simulink model "BLAC_MotorCtrl_Math"  (R2023b)
settings: Solver=FixedStepDiscrete  StartTime=0.0  StopTime=0.1  FixedStep=MC_Sim_BaseStep  RelTol=1e-3  EnableMultiTasking=on
values from neighbouring files (symbols this model uses):
  MC_Hardware_Chip_ADCResultBit = 0.0    [MotorControlDataDictionary_Math.sldd]
  MC_Hardware_Chip_ADCVoltageMax = 1.0    [MotorControlDataDictionary_Math.sldd]
  MC_Hardware_Chip_ADCVoltageRefence = 0.0    [MotorControlDataDictionary_Math.sldd]
  MC_Hardware_Chip_CSAGain = 1.0    [MotorControlDataDictionary_Math.sldd]
  MC_Hardware_Sample_Resistor = 0.001    [MotorControlDataDictionary_Math.sldd]
  MC_MotorModel_Machine_Damp = 0.0    [MotorControlDataDictionary_Math.sldd]
  MC_MotorModel_Machine_Ineria = 0.0    [MotorControlDataDictionary_Math.sldd]
  MC_MotorModel_Machine_Tfric = 0.0    [MotorControlDataDictionary_Math.sldd]
  MC_MotorModel_Rotor_Pn = 4.0    [MotorControlDataDictionary_Math.sldd]
  MC_MotorModel_Stator_Ld = 0.0    [MotorControlDataDictionary_Math.sldd]
  MC_MotorModel_Stator_Lq = 0.0    [MotorControlDataDictionary_Math.sldd]
  MC_MotorModel_Stator_Rs = 1.0    [MotorControlDataDictionary_Math.sldd]
  MC_Sim_BaseStep = 2.5E-8    [MotorControlDataDictionary_Math.sldd]
  MC_Sim_HFTStep = 6.6675E-5    [MotorControlDataDictionary_Math.sldd]
undefined symbols (not defined in the file or in its folder): MC_MOS_DeadTime, MC_Motor_Phi, MC_Motor_Rotor_Pn, MC_Motor_Stator_Ld, MC_Motor_Stator_Lq, MC_Motor_Stator_Rs, MC_Param_CurrentPI_Ki, MC_Param_CurrentPI_Kp, MC_Param_CurrentPI_UdInteMax, MC_Param_CurrentPI_UdInteMin, MC_Param_CurrentPI_UdMax, MC_Param_CurrentPI_UdMin, MC_Param_CurrentPI_UqInteMax, MC_Param_CurrentPI_UqInteMin, MC_Param_CurrentPI_UqMax, MC_Param_CurrentPI_UqMin, MC_Param_Flux_Gamma, MC_Param_Flux_Lalpha, MC_Param_Flux_Lbeta, MC_Param_Flux_Ralpha, MC_Param_Flux_Rbeta, MC_Param_Luen_BEMFalpha, MC_Param_Luen_BEMFbeta, MC_Param_Luen_BEMFErr, MC_Param_Luen_Currentalpha, MC_Param_Luen_Currentbeta, MC_Param_Luen_CurrentErr, MC_Param_Luen_PLL_Ki, MC_Param_Luen_PLL_Kp, MC_Param_Luen_Voltagealpha, MC_Param_Luen_Voltagebeta, MC_Param_PhasetoReal, MC_Param_SMO_CoffA, MC_Param_SMO_CoffB, MC_Param_SpeedtoTheta, MC_Param_SVPWM_DutyMax, MC_Param_SVPWM_DutyMin, MC_Param_SVPWM_SampleOffset1, MC_Param_SVPWM_SampleOffset2, MC_Param_SVPWM_SampleValid
libraries: simulink x29, spsSeriesRLCBranchLib x6, spsVoltageMeasurementLib x6, spsIGBTLib x6, spsDiodeLib x4, spsACVoltageSourceLib x1, spsGroundLib x1, spsPermanentMagnetSynchronousMachineLib x1, spsThreePhaseVIMeasurementLib x1, spspowerguiLib x1
(part 1 of 3)
settings Model: DataDictionary=MotorControlDataDictionary_Math.sldd  SimulationMode=accelerator  Creator=YXuan  LastModifiedBy=YXuan
settings SolverCC: PositivePriorityOrder=on
settings OptimizationCC: DefaultParameterBehavior=Inlined  EnhancedBackFolding=on  PassReuseOutputArgsAs=Individual arguments  ZeroExternalMemoryAtStartup=off  ZeroInternalMemoryAtStartup=off  OptimizeBlockOrder=speed  DifferentSizesBufferReuse=on  OptimizationCustomize=off  EfficientTunableParamExpr=on
settings DebuggingCC: ParameterTunabilityLossMsg=error
settings SFSimCC: MATLABDynamicMemAlloc=off
settings RTWCC: Description=Embedded Coder  SystemTargetFile=ert.tlc  TemplateMakefile=ert_default_tmf
settings CodeAppCC: ForceParamTrailComments=on  IgnoreCustomStorageClasses=off  OperatorAnnotations=on  SimulinkDataObjDesc=on  SFDataObjDesc=on  InsertBlockDesc=on
settings ERTTargetCC: TargetLangStandard=C99 (ISO)  GenerateSampleERTMain=on  InlinedParameterPlacement=NonHierarchical  ERTCustomFileTemplate=example_file_process.tlc

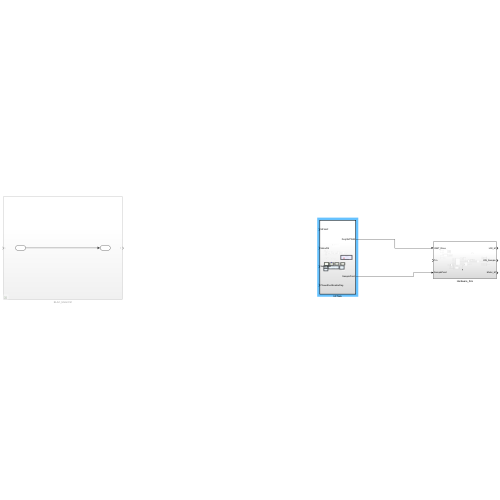
[thumbnail: Simulink's stored preview of the top-level diagram]
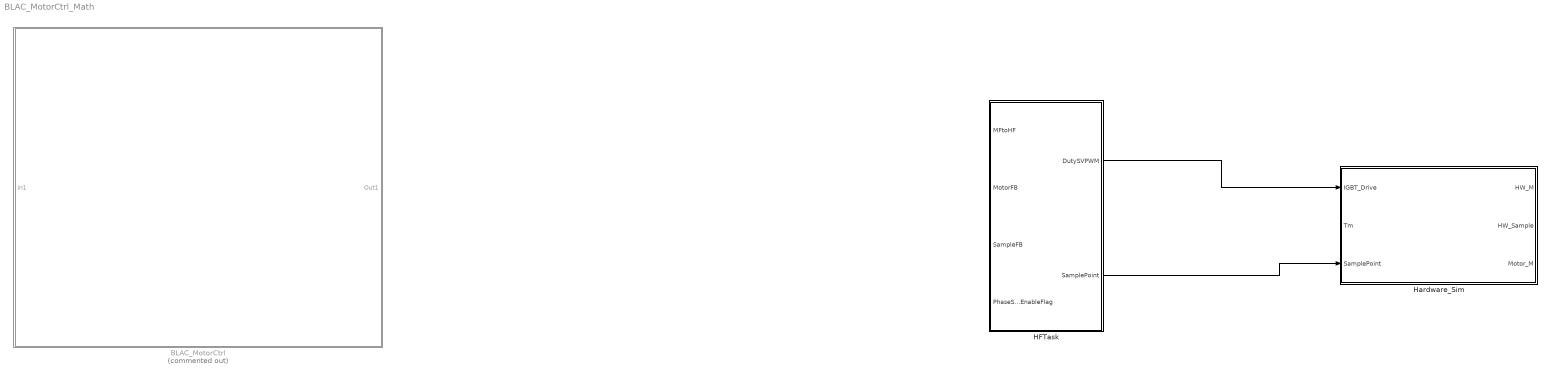
== system BLAC_MotorCtrl_Math ==
  BLAC_MotorCtrl : Subsystem  Commented=on
  HFTask : Subsystem  TreatAsAtomicUnit=on  SystemSampleTime=MC_Sim_HFTStep
  Hardware_Sim : Subsystem
  wires:
  HFTask/1(DutySVPWM) -> Hardware_Sim/1(IGBT_Drive)
  HFTask/2(SamplePoint) -> Hardware_Sim/3(SamplePoint)

== system BLAC_MotorCtrl_Math/BLAC_MotorCtrl ==
  In1 : Inport
  Out1 : Outport
  wires:
  In1/1 -> Out1/1

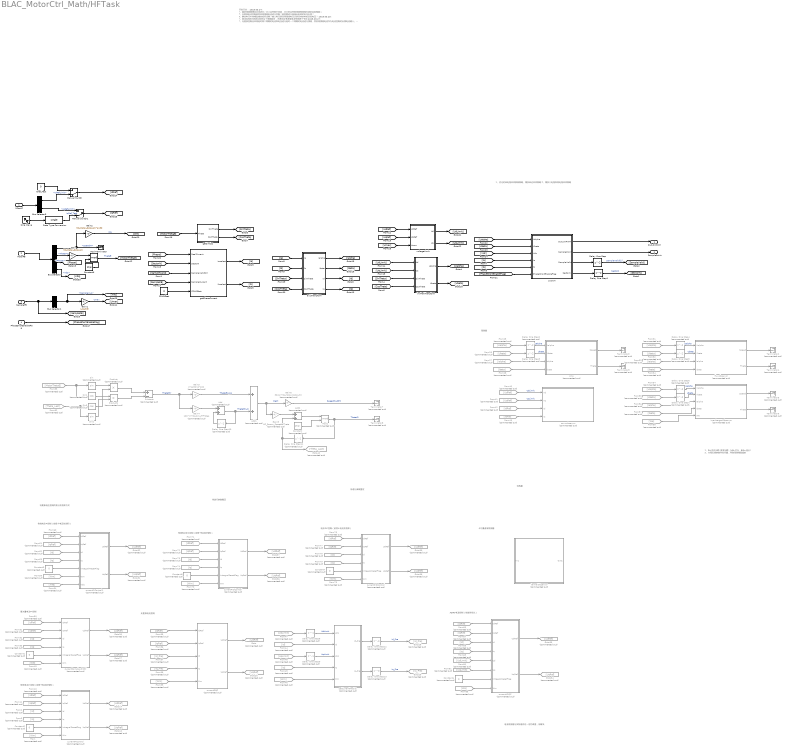
== system BLAC_MotorCtrl_Math/HFTask ==
  note: 待更新电压控制的积分抗饱和方式
  note: 传统电流PI控制（前馈+电流抗饱和）
  note: 1、PLL存在问题(带宽问题，10hz可以，50hz溢出)
      | 2、方程反馈参数存在问题，导致观测角度超前
  note: 观测器
  note: 无差拍电流控制
  note: 开发日志：
      | 2025.03.24:
      | 1、磁链观测器增益应该适中（过小会导致不收敛，过大则会导致观测角度相位超前实际角度）
      | 2、无差拍电流控制是否采用预测电流进行控制？是否要进行旋转反电势的电压补偿？
      | 3、静态电压补偿模型增益如何设置？输入电压是采用理想电压还是采样的电机实际电压？
      | 2025.03.25:
      | 1、测试发现电压和电流呈现2个周期延时，无差拍应考虑做电流预测两个节拍
      | 2025.03.27：
      | 1、无差拍控制应采用延时两个周期的电流和电压进行延时一个周期的电流进行预测，然后用预测电流作为电流控制的反馈电流输入。
      | 2025.12.13:
      | 1、增加真实相电压计算（待添加）
      | 2、考虑MPTA、弱磁、以及MPTV模块的防止位置
      | 2026.01.01：
      | 1、增加卡尔曼滤波模块（未构建）
      | 2、增加PIR控制器（未整定参数）
      | 2026.01.28：
      | 1、发现ADRC的电流观测值初期收敛速度较慢，并且存在稳定的误差。
  note: 复矢量电流PI控制
  note: 传统电流PI控制（前馈+电压抗饱和）
  note: ADRC电流控制（性能待优化）
  note: 传统电流PID控制（前馈+电流抗饱和）
  note: 待进行参数整定
  note: 电流PIR控制（前馈+电流抗饱和）
  note: 待进行参数整定
  note: 卡尔曼滤波观测器
  note: 待构建
  note: 1、优化的单电阻采样移相策略、增加单边采样策略
      | 2、增加三电阻和两电阻采样策略
  note: 电流观测值与实际值存在一定的误差，待解决
  MFtoHF : Inport
  MotorFB : Inport  Port=2
  SampleFB : Inport  Port=3
  PhaseShortEnableFlag : Inport  Port=4
  Add : Sum  Commented=on
  Add1 : Sum  Commented=on
  Add2 : Sum  Commented=on
  Bus Selector : BusSelector  OutputSignals=SpeedM,ThetaM,PhaseI,Vdq
  Bus Selector1 : BusSelector  OutputSignals=SampleVus
  Bus Selector3 : BusSelector  OutputSignals=IdRefLimit,IqRefLimit
  CSAOffset : Constant  Value=0  OutDataTypeStr=single
  Constant : Constant  Commented=on  Value=2*pi  OutDataTypeStr=single
  Constant{1..5,7} (6 alike) : Constant  Commented=on  Value=0  OutDataTypeStr=boolean
  Constant6 : Constant  Value=2*pi  OutDataTypeStr=single
  Data Type Conversion : DataTypeConversion  OutDataTypeStr=single  RndMeth=Simplest  SaturateOnIntegerOverflow=off
  Delay One Step : Delay
  Delay One Step1 : Delay
  Delay One Step{8..11} (4 alike) : Delay  Commented=on  DelayLength=1
  Delay One Step12 : Delay  Commented=on  DelayLength=0
  Delay One Step13 : Delay  Commented=on  DelayLength=0
  Delay One Step{2..7} (6 alike) : Delay  Commented=on
  From{,39,46,59,70,75} (6 alike) : From  Commented=on  GotoTag=Wm
  From{10,35,42,50,60,66,71,76} (8 alike) : From  Commented=on  GotoTag=IdRef
  From{11,36,43,51,61,67,72,77} (8 alike) : From  Commented=on  GotoTag=IqRef
  From{2,44,52,62,68,73,78} (7 alike) : From  Commented=on  GotoTag=Id
  From25 : From  Commented=on  GotoTag=Ualpha
  From26 : From  Commented=on  GotoTag=Ubeta
  From27 : From  Commented=on  GotoTag=Ialpha
  From28 : From  Commented=on  GotoTag=Ibeta
  From{3,45,53,63,69,74,79} (7 alike) : From  Commented=on  GotoTag=Iq
  From31 : From  Commented=on  GotoTag=Ualpha
  From32 : From  Commented=on  GotoTag=Ubeta
  From33 : From  Commented=on  GotoTag=Ialpha
  From34 : From  Commented=on  GotoTag=Ibeta
  From37 : From  Commented=on  GotoTag=Id_Pre
  From38 : From  Commented=on  GotoTag=Iq_Pre
  From40 : From  Commented=on  GotoTag=UdRef
  From41 : From  Commented=on  GotoTag=UqRef
  From47 : From  Commented=on  GotoTag=UdLimit
  From48 : From  Commented=on  GotoTag=UqLimit
  From49 : From  Commented=on  GotoTag=We
  From54 : From  Commented=on  GotoTag=Ualpha
  From55 : From  Commented=on  GotoTag=Ubeta
  From56 : From  Commented=on  GotoTag=Ialpha
  From57 : From  Commented=on  GotoTag=Ibeta
  From58 : From  Commented=on  GotoTag=We
  From64 : From  Commented=on  GotoTag=Vdq
  From65 : From  Commented=on  GotoTag=We
  From80 : From  Commented=on  GotoTag=UdLimit
  From81 : From  Commented=on  GotoTag=UqLimit
  From82 : From  Commented=on  GotoTag=Theta_Last
  From83 : From  Commented=on  GotoTag=MotorThetaE
  Gain : Gain  Gain=MC_Motor_Rotor_Pn  OutDataTypeStr=single
  Gain1 : Gain  Gain=1/sqrt(3)  OutDataTypeStr=single
  Gain2 : Gain  Gain=MC_Motor_Rotor_Pn*pi/30
  Gain3 : Gain  Commented=on  Gain=2*sqrt(2)/2*100
  Gain4 : Gain  Commented=on  Gain=100^2*MC_Sim_HFTStep
  Gain5 : Gain  Commented=on  Gain=MC_Param_SpeedtoTheta  OutDataTypeStr=single  RndMeth=Simplest
  Gain6 : Gain  Commented=on  Gain=30/(pi*MC_Motor_Rotor_Pn)  OutDataTypeStr=single  RndMeth=Simplest
  Goto{,14,30,32,35,37,39} (7 alike) : Goto  Commented=on  GotoTag=UdRef
  Goto{10,26..27,31,34,36,38} (7 alike) : Goto  Commented=on  GotoTag=UqRef
  Goto28 : Goto  Commented=on  GotoTag=Id_Pre
  Goto29 : Goto  Commented=on  GotoTag=Iq_Pre
  Goto40 : Goto  Commented=on  GotoTag=Theta_Last
  Idref_Test : Constant  Value=0  OutDataTypeStr=single
  LuenbergerObservor : Subsystem  Commented=on
  Manual Switch : ManualSwitch  CurrentSetting=0
  Manual Switch1 : ManualSwitch  CurrentSetting=0
  Mod : Math  Operator=mod
  Mod1 : Math  Commented=on  Operator=mod
  Product : Product  Commented=on
  Product1 : Product  Commented=on
  Sin : Trigonometry  Commented=on  OutputSignalType=real
  Sin1 : Trigonometry  Commented=on  Operator=cos  OutputSignalType=real
  Sin2 : Trigonometry  Commented=on  OutputSignalType=real
  Sin3 : Trigonometry  Commented=on  Operator=cos  OutputSignalType=real
  Sine Wave : Sin  Amplitude=20  Frequency=2*pi*1  SampleTime=MC_Sim_HFTStep
  Subtract : Sum  Commented=on  Inputs=+-
  Terminator : Terminator
  Terminator{1..8} (8 alike) : Terminator  Commented=on
  axisTransform : Subsystem
  currentADRC : Subsystem  Commented=on
  currentComplexPICtrl : Subsystem  Commented=on
  currentDBC : Subsystem  Commented=on
  currentPIControl : Subsystem  Commented=on
  currentPIControl1 : Subsystem  Commented=on
  currentPIDControl : Subsystem  Commented=on
  currentPIRControl : Subsystem  Commented=on
  fluxobservor : Subsystem  Commented=on
  getCurrentPredict : Subsystem  Commented=on
  getPhaseCurrent : Subsystem
  getSinCos : Subsystem
  invParkTransform : Subsystem
  karmalObservor : Subsystem  Commented=on
  scvmobservor : Subsystem  Commented=on
  smo : Subsystem  Commented=on
  svpwm : Subsystem  TreatAsAtomicUnit=on
  voltageLimit : Subsystem
  DutySVPWM : Outport
  SamplePoint : Outport  Port=2
  wires:
  MFtoHF/1 -> Bus Selector3/1
  Delay One Step2/1 -> smo/1(Valpha)  "Ualpha"
  From25/1 -> Delay One Step2/1
  Delay One Step3/1 -> smo/2(Vbeta)  "Ubeta"
  From26/1 -> Delay One Step3/1
  From27/1 -> smo/3(Ialpha)
  From28/1 -> smo/4(Ibeta)
  smo/1(Speed) -> Terminator2/1
  smo/2(Theta) -> Terminator3/1
  [PhaseShortEnableFlag] -> svpwm/6(PhaseShortEnableFlag)
  [Umax] -> voltageLimit/3(Umax)
  svpwm/4(SectorN) -> Delay One Step1/1
  axisTransform/2(Ibeta) -> [Ibeta]
  svpwm/3(SampleValid) -> Delay One Step/1
  svpwm/1(DutySVPWM) -> DutySVPWM/1
  [SampleFB] -> getPhaseCurrent/4(SampleCurrent)
  [SectorN] -> getPhaseCurrent/2(SectorN)
  [UdRef] -> voltageLimit/1(UdRef)
  [UdLimit] -> invParkTransform/1(Ud)
  currentPIControl/1(UdRef) -> Goto14/1
  [Ubeta] -> svpwm/2(Vbeta)
  axisTransform/1(Ialpha) -> [Ialpha]
  [UqRef] -> voltageLimit/2(UqRef)
  [Ualpha] -> svpwm/1(Valpha)
  [Ia] -> axisTransform/1(Ia)
  svpwm/2(SamplePoint) -> SamplePoint/1
  currentPIControl/2(UqRef) -> Goto10/1
  [Vdc] -> svpwm/3(Vdc)
  voltageLimit/1(Ud) -> [UdLimit]
  [MotorThetaE] -> getSinCos/1(Theta)
  From2/1 -> currentPIControl/3(Id)
  getSinCos/1(SinTheta) -> [SinTheta]
  [SampleValid] -> getPhaseCurrent/3(SampleValid[2])
  axisTransform/3(Id) -> [Id]
  getPhaseCurrent/2(Ibselect) -> [Ib]
  From/1 -> currentPIControl/6(Wm)
  axisTransform/4(Iq) -> [Iq]
  From3/1 -> currentPIControl/4(Iq)
  Constant2/1 -> currentPIControl/5(IntregralResetFlag)
  [Ib] -> axisTransform/2(Ib)
  [UqLimit] -> invParkTransform/2(Uq)
  [SinTheta] -> invParkTransform/3(SinTheta)
  Delay One Step1/1 -> [SectorN]  "SectorN"
  [CosTheta] -> invParkTransform/4(CosTheta)
  [PhaseI] -> getPhaseCurrent/1(RealCurrent)
  invParkTransform/1(Ualpha) -> [Ualpha]
  Delay One Step/1 -> [SampleValid]  "SampleValid[2]"
  getSinCos/2(CosTheta) -> [CosTheta]
  voltageLimit/2(Uq) -> [UqLimit]
  [SinTheta] -> axisTransform/3(SinTheta)
  getPhaseCurrent/1(Iaselect) -> [Ia]
  CSAOffset/1 -> getPhaseCurrent/5(CSAOffset)
  [CosTheta] -> axisTransform/4(CosTheta)
  invParkTransform/2(Ubeta) -> [Ubeta]
  [Ib] -> svpwm/5(Ib)
  [Ia] -> svpwm/4(Ia)
  Bus Selector/2 -> Gain/1  "<ThetaM>"
  PhaseShortEnableFlag/1 -> [PhaseShortEnableFlag]
  Bus Selector/1 -> Terminator/1, Gain2/1  "<SpeedM>"
  Mod/1 -> [MotorThetaE]  "ThetaE"
  Bus Selector/3 -> [PhaseI]  "<PhaseI>"
  Gain/1 -> Mod/1
  Bus Selector1/1 -> [Vdc], Gain1/1  "<SampleVus>"
  SampleFB/1 -> [SampleFB], Bus Selector1/1
  Gain1/1 -> [Umax]  "Umax"
  Constant6/1 -> Mod/2
  MotorFB/1 -> Bus Selector/1
  From10/1 -> currentPIControl/1(IdRef)
  From11/1 -> currentPIControl/2(IqRef)
  From34/1 -> fluxobservor/4(Ibeta)
  From33/1 -> fluxobservor/3(Ialpha)
  From32/1 -> Delay One Step5/1
  From31/1 -> Delay One Step4/1
  Delay One Step4/1 -> fluxobservor/1(Valpha)  "Ualpha"
  Delay One Step5/1 -> fluxobservor/2(Vbeta)  "Ubeta"
  fluxobservor/1(Speed) -> Terminator1/1
  fluxobservor/2(Theta) -> Terminator4/1
  currentDBC/2(UqRef) -> Goto26/1
  From36/1 -> currentDBC/2(IqRef)
  From35/1 -> currentDBC/1(IdRef)
  From37/1 -> currentDBC/3(Id)
  From38/1 -> currentDBC/4(Iq)
  From39/1 -> currentDBC/5(Wm)
  From41/1 -> scvmobservor/2(Vq)  "UqLimit"
  From40/1 -> scvmobservor/1(Vd)  "UdLimit"
  From42/1 -> scvmobservor/3(Id)
  From43/1 -> scvmobservor/4(Iq)
  Gain2/1 -> [We]  "We"
  From44/1 -> getCurrentPredict/2(Id)
  From45/1 -> getCurrentPredict/4(Iq)
  From46/1 -> getCurrentPredict/5(Wm)
  From47/1 -> Delay One Step8/1
  From48/1 -> Delay One Step9/1
  getCurrentPredict/1(Id_Pre) -> Delay One Step12/1
  getCurrentPredict/2(Iq_Pre) -> Delay One Step13/1
  currentDBC/1(UdRef) -> Goto/1
  Delay One Step8/1 -> getCurrentPredict/1(Ud1)  "UdLimit"
  Delay One Step9/1 -> getCurrentPredict/3(Uq1)  "UqLimit"
  Delay One Step12/1 -> Goto28/1  "Id_Pre"
  Delay One Step13/1 -> Goto29/1  "Iq_Pre"
  From51/1 -> currentComplexPICtrl/2(IqRef)
  From50/1 -> currentComplexPICtrl/1(IdRef)
  Constant1/1 -> currentComplexPICtrl/5(IntregralResetFlag)
  From53/1 -> currentComplexPICtrl/4(Iq)
  From49/1 -> currentComplexPICtrl/6(Wm)
  From52/1 -> currentComplexPICtrl/3(Id)
  currentComplexPICtrl/2(UqRef) -> Goto27/1
  currentComplexPICtrl/1(UdRef) -> Goto30/1
  LuenbergerObservor/1(Speed) -> Terminator5/1
  LuenbergerObservor/2(Theta) -> Terminator6/1
  From57/1 -> LuenbergerObservor/4(Ibeta)
  From56/1 -> LuenbergerObservor/3(Ialpha)
  From55/1 -> Delay One Step7/1
  From54/1 -> Delay One Step6/1
  Delay One Step7/1 -> LuenbergerObservor/2(Vbeta)  "Ubeta"
  Delay One Step6/1 -> LuenbergerObservor/1(Valpha)  "Ualpha"
  From58/1 -> LuenbergerObservor/5(We)
  From61/1 -> currentPIControl1/2(IqRef)
  From60/1 -> currentPIControl1/1(IdRef)
  Constant3/1 -> currentPIControl1/5(IntregralResetFlag)
  From63/1 -> currentPIControl1/4(Iq)
  From59/1 -> currentPIControl1/6(Wm)
  From62/1 -> currentPIControl1/3(Id)
  currentPIControl1/2(UqRef) -> Goto31/1
  currentPIControl1/1(UdRef) -> Goto32/1
  Bus Selector/4 -> [Vdq]  "<Vdq>"
  From64/1 -> currentPIControl1/7(Vdq)
  currentADRC/1(UdRef) -> Goto35/1
  currentADRC/2(UqRef) -> Goto34/1
  From68/1 -> currentADRC/3(Id)
  From65/1 -> currentADRC/8(Wm)
  From69/1 -> currentADRC/4(Iq)
  Constant4/1 -> currentADRC/7(IntregralResetFlag)
  From66/1 -> currentADRC/1(IdRef)
  From67/1 -> currentADRC/2(IqRef)
  Constant5/1 -> currentPIDControl/5(IntregralResetFlag)
  From71/1 -> currentPIDControl/1(IdRef)
  currentPIDControl/1(UdRef) -> Goto37/1
  From73/1 -> currentPIDControl/3(Id)
  From72/1 -> currentPIDControl/2(IqRef)
  currentPIDControl/2(UqRef) -> Goto36/1
  From70/1 -> currentPIDControl/6(Wm)
  From74/1 -> currentPIDControl/4(Iq)
  Bus Selector3/1 -> Manual Switch/2  "<IdRefLimit>"
  Bus Selector3/2 -> Manual Switch1/1  "<IqRefLimit>"
  Sine Wave/1 -> Data Type Conversion/1
  Manual Switch/1 -> [IdRef]
  Idref_Test/1 -> Manual Switch/1
  Manual Switch1/1 -> [IqRef]
  Data Type Conversion/1 -> Manual Switch1/2  "IqRef_Test"
  From79/1 -> currentPIRControl/4(Iq)
  From75/1 -> currentPIRControl/6(Wm)
  currentPIRControl/2(UqRef) -> Goto38/1
  From77/1 -> currentPIRControl/2(IqRef)
  From78/1 -> currentPIRControl/3(Id)
  currentPIRControl/1(UdRef) -> Goto39/1
  From76/1 -> currentPIRControl/1(IdRef)
  Constant7/1 -> currentPIRControl/5(IntregralResetFlag)
  From80/1 -> currentADRC/5(Ud)
  From81/1 -> currentADRC/6(Uq)
  Gain5/1 -> Add2/1
  Delay One Step10/1 -> Add/2
  Constant/1 -> Mod1/2
  Mod1/1 -> Terminator8/1, Delay One Step11/1  "ThetaPI"
  Delay One Step11/1 -> Goto40/1, Add2/2
  Gain3/1 -> Add1/1  "ThetaErr_Kp"
  Add1/1 -> Gain6/1, Gain5/1  "WePI"
  Add2/1 -> Mod1/1
  Gain6/1 -> Terminator7/1  "SpeedPI_RPM"
  Subtract/1 -> Gain3/1, Gain4/1  "ThetaErr"
  Add/1 -> Add1/2, Delay One Step10/1  "ThetaErr_Ki"
  Gain4/1 -> Add/1
  From83/1 -> Sin1/1, Sin/1
  From82/1 -> Sin2/1, Sin3/1
  Sin/1 -> Product/1
  Sin3/1 -> Product/2
  Product/1 -> Subtract/1
  Sin1/1 -> Product1/1
  Sin2/1 -> Product1/2
  Product1/1 -> Subtract/2

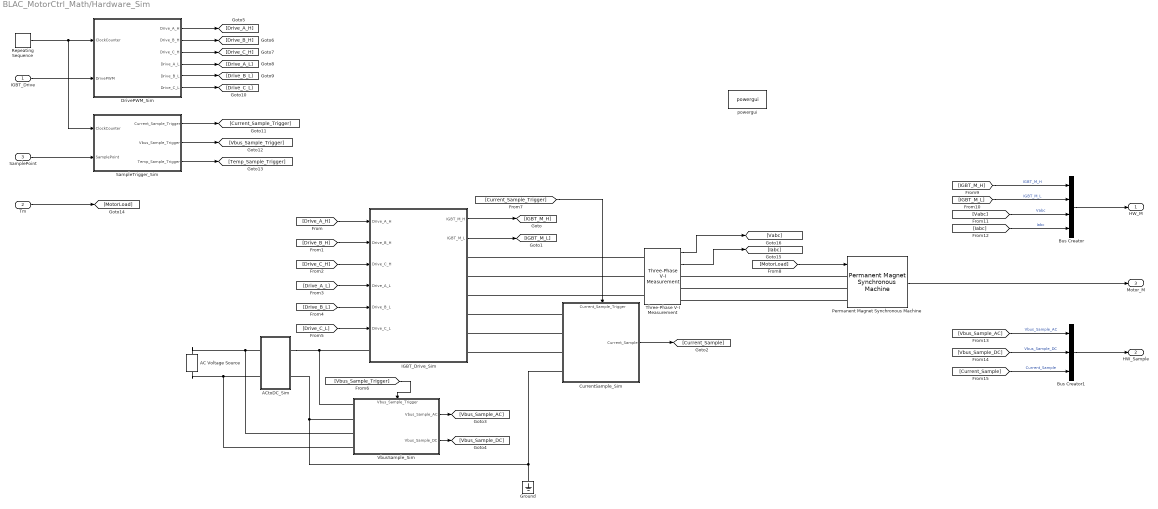
== system BLAC_MotorCtrl_Math/Hardware_Sim ==
  IGBT_Drive : Inport
  Tm : Inport  Port=2
  SamplePoint : Inport  Port=3
  AC Voltage Source : spsACVoltageSourceLib/AC Voltage Source  Amplitude=220*sqrt(2)  Phase=0  Frequency=50  SampleTime=-1  Measurements=None  BusType=swing  Pref=10e3  Qref=0  Qmin=-inf  Qmax=+inf
  ACtoDC_Sim : Subsystem
  Bus Creator : BusCreator  Inputs=4
  Bus Creator1 : BusCreator  Inputs=3
  CurrentSample_Sim : Subsystem
      settings: PortSchema="{\"entries\":[{\"content\":{\"sides\":[{\"content\":{\"connectorIds\":[\"LConn1\",\"LConn2\",\"LConn3\",\"LConn4\"]},\"type\":\"ConnectorPlacement.EquallySpacedRectSide\",\"uuid\":\"6ff7a8d3-c405-46c2-bb14-4046cb7aeae7\"},{\"content\":{\"connectorIds\":[\"Out1\"],\"side\":\"RIGHT\"},\"type\":\"ConnectorPlacement.EquallySpacedRectSide\",\"uuid\":\"30142a9b-9a7e-41fc-b1d2-e3039139c6ca\"},{\"content\":{\"connectorIds\":[\"In1\"],\"side\":\"TOP\"},\"type\":\"ConnectorPlacement.EquallySpacedRectSide\",\"uuid\":\"3160108e-a18c-4d1a-9078-164fb8c05fb9\"}]},\"type\":\"ConnectorPlacement.EquallySpacedConnector\",\"uuid\":\"b4e632a6-7f3d-4ba3-a4f0-ad8004e8ab56\"}],\"packageUris\":[\"http://schema.mathworks.com/mf0/Connector/R2020b\"],\"version\":\"1.0\"}"
  DrivePWM_Sim : Subsystem
  Ground : spsGroundLib/Ground  LConnTagsString=a
  IGBT_Drive_Sim : Subsystem
  Permanent Magnet Synchronous Machine : spsPermanentMagnetSynchronousMachineLib/Permanent Magnet Synchronous Machine  NbPhases=3  FluxDistribution=Sinusoidal  RotorType=Salient-pole  MechanicalLoad=Torque Tm  PresetModel=No  ShowDetailedParameters=on  MeasurementBus=on  Resistance=MC_MotorModel_Stator_Rs  Inductance=8.5e-3  dqInductances=[MC_MotorModel_Stator_Ld,MC_MotorModel_Stator_Lq]  La=0.000395  MachineConstant=Voltage Constant (V_peak L-L / krpm)  Flux=0  VoltageCst=MC_MotorModel_Magentic_Ke  TorqueCst=0  Flat=120  Mechanical=[MC_MotorModel_Machine_Ineria,MC_MotorModel_Machine_Damp,MC_MotorModel_Rotor_Pn,MC_MotorModel_Machine_Tfric]  PolePairs=4  InitialConditions=[0,0, 0,0]  InitialConditions5ph=[0 0 0 0 0 0]  RefAngle=Aligned with phase A axis (original Park)  IterativeDiscreteModel=Trapezoidal non iterative  TsBlock=-1  TsPowergui=0
  Repeating Sequence : simulink/Sources/Repeating Sequence  rep_seq_t=[0 MC_Sim_HFTStep/2 MC_Sim_HFTStep]  rep_seq_y=[0 1 0]
  SampleTrigger_Sim : Subsystem
  Three-Phase V-I Measurement : spsThreePhaseVIMeasurementLib/Three-Phase V-I Measurement  VoltageMeasurement=phase-to-ground  SetLabelV=off  LabelV=Vabc  Vpu=off  VpuLL=off  CurrentMeasurement=yes  SetLabelI=off  LabelI=Iabc  Ipu=off  Pbase=100e6  Vbase=500e3  OutputType=Complex  PhasorSimulation=off  PSBequivalent=0
  VbusSample_Sim : Subsystem
      settings: PortSchema="{\"entries\":[{\"content\":{\"sides\":[{\"content\":{\"connectorIds\":[\"LConn1\",\"LConn2\",\"LConn3\",\"LConn4\"]},\"type\":\"ConnectorPlacement.EquallySpacedRectSide\",\"uuid\":\"516f667a-d28d-4d7e-bf09-1844ec397ca8\"},{\"content\":{\"connectorIds\":[\"Out1\",\"Out2\"],\"side\":\"RIGHT\"},\"type\":\"ConnectorPlacement.EquallySpacedRectSide\",\"uuid\":\"8e4c85e3-3d11-4eb4-88a0-2693c28d829e\"},{\"content\":{\"connectorIds\":[\"In1\"],\"side\":\"TOP\"},\"type\":\"ConnectorPlacement.EquallySpacedRectSide\",\"uuid\":\"147b6efa-5ce1-4794-b48d-7dda172e67f0\"}]},\"type\":\"ConnectorPlacement.EquallySpacedConnector\",\"uuid\":\"ecacdeaf-2c45-44a5-a2ad-63e6b49d0bd0\"}],\"packageUris\":[\"http://schema.mathworks.com/mf0/Connector/R2020b\"],\"version\":\"1.0\"}"
  powergui : spspowerguiLib/powergui  Priority=1  SimulationMode=Discrete  SampleTime=MC_Sim_BaseStep  frequency=60  Iterations=50  frequencyindice=50  Pbase=100e6  ErrMax=1e-4  UnitsV=kV  UnitsW=MW  buscounter=0  FunctionMessages=off  echomessages=off  EnableUseOfTLC=off  CurrentSourceSwitches=off  DisableSnubberDevices=off  DisableRonSwitches=off  DisableVfSwitches=off  DisplayEquations=off  AutomaticDiscreteSolvers=off  SolverType=Tustin/Backward Euler (TBE)  Interpol=off  ExternalGateDelay=off  methode=off  Ts=100  x0status=blocks  SPID=on  SwTol=0  HookPort=off  NonlinearTolerance=1e-4  nMaxIteration=100  ContinueOnMaxIteration=off  RestoreLinks=warning  ResistiveCurrentMeasurement=off  Frange=[0:2:500]  Ylog=off  Xlog=on  ShowGrid=off  save=off  variable=ZData  structure=0  ZoomFFT=off  StartTime=0.0  cycles=1  DisplayStyle=1  fundamental=60  FreqAxis=off  MaxFrequency=1000  frequencyindicesteady=1  RmsSteady=1  display=off
  HW_M : Outport
  HW_Sample : Outport  Port=2
  Motor_M : Outport  Port=3
  wires:
  Permanent Magnet Synchronous Machine/1 -> Motor_M/1
  IGBT_Drive_Sim/1(IGBT_M_H) -> [IGBT_M_H]
  IGBT_Drive_Sim/2(IGBT_M_L) -> [IGBT_M_L]
  CurrentSample_Sim/1(Current_Sample) -> [Current_Sample]
  VbusSample_Sim/1(Vbus_Sample_AC) -> [Vbus_Sample_AC]
  VbusSample_Sim/2(Vbus_Sample_DC) -> [Vbus_Sample_DC]
  SamplePoint/1 -> SampleTrigger_Sim/2(SamplePoint)
  Repeating Sequence/1 -> SampleTrigger_Sim/1(ClockCounter), DrivePWM_Sim/1(ClockCounter)
  IGBT_Drive/1 -> DrivePWM_Sim/2(DrivePWM)
  DrivePWM_Sim/1(Drive_A_H) -> [Drive_A_H]
  DrivePWM_Sim/2(Drive_B_H) -> [Drive_B_H]
  DrivePWM_Sim/6(Drive_C_L) -> [Drive_C_L]
  DrivePWM_Sim/5(Drive_B_L) -> [Drive_B_L]
  DrivePWM_Sim/4(Drive_A_L) -> [Drive_A_L]
  DrivePWM_Sim/3(Drive_C_H) -> [Drive_C_H]
  SampleTrigger_Sim/1(Current_Sample_Trigger) -> [Current_Sample_Trigger]
  SampleTrigger_Sim/2(Vbus_Sample_Trigger) -> [Vbus_Sample_Trigger]
  SampleTrigger_Sim/3(Temp_Sample_Trigger) -> [Temp_Sample_Trigger]
  [Drive_A_H] -> IGBT_Drive_Sim/1(Drive_A_H)
  [Drive_B_H] -> IGBT_Drive_Sim/2(Drive_B_H)
  [Drive_C_H] -> IGBT_Drive_Sim/3(Drive_C_H)
  [Drive_A_L] -> IGBT_Drive_Sim/4(Drive_A_L)
  [Drive_B_L] -> IGBT_Drive_Sim/5(Drive_B_L)
  [Drive_C_L] -> IGBT_Drive_Sim/6(Drive_C_L)
  [Vbus_Sample_Trigger] -> VbusSample_Sim/1(Vbus_Sample_Trigger)
  Tm/1 -> [MotorLoad]
  [MotorLoad] -> Permanent Magnet Synchronous Machine/1
  [Current_Sample_Trigger] -> CurrentSample_Sim/1(Current_Sample_Trigger)
  Three-Phase V-I Measurement/2 -> [Iabc]
  Three-Phase V-I Measurement/1 -> [Vabc]
  [IGBT_M_H] -> Bus Creator/1  "IGBT_M_H"
  [IGBT_M_L] -> Bus Creator/2  "IGBT_M_L"
  [Vabc] -> Bus Creator/3  "Vabc"
  [Iabc] -> Bus Creator/4  "Iabc"
  [Vbus_Sample_AC] -> Bus Creator1/1  "Vbus_Sample_AC"
  [Current_Sample] -> Bus Creator1/3  "Current_Sample"
  [Vbus_Sample_DC] -> Bus Creator1/2  "Vbus_Sample_DC"
  Bus Creator/1 -> HW_M/1
  Bus Creator1/1 -> HW_Sample/1
  connections:
  Permanent Magnet Synchronous Machine/LConn2 -- Three-Phase V-I Measurement/RConn2
  Permanent Magnet Synchronous Machine/LConn1 -- Three-Phase V-I Measurement/RConn1
  Permanent Magnet Synchronous Machine/LConn3 -- Three-Phase V-I Measurement/RConn3
  AC Voltage Source/RConn1 -- VbusSample_Sim/LConn3 -- ACtoDC_Sim/LConn1
  AC Voltage Source/LConn1 -- VbusSample_Sim/LConn4 -- ACtoDC_Sim/LConn2
  ACtoDC_Sim/RConn1 -- IGBT_Drive_Sim/LConn1 -- VbusSample_Sim/LConn1
  VbusSample_Sim/LConn2 -- Ground/LConn1 -- CurrentSample_Sim/LConn4 -- ACtoDC_Sim/RConn2
  CurrentSample_Sim/LConn1 -- IGBT_Drive_Sim/RConn4
  CurrentSample_Sim/LConn2 -- IGBT_Drive_Sim/RConn5
  CurrentSample_Sim/LConn3 -- IGBT_Drive_Sim/RConn6
  Three-Phase V-I Measurement/LConn1 -- IGBT_Drive_Sim/RConn1
  Three-Phase V-I Measurement/LConn2 -- IGBT_Drive_Sim/RConn2
  Three-Phase V-I Measurement/LConn3 -- IGBT_Drive_Sim/RConn3

== system BLAC_MotorCtrl_Math/HFTask/LuenbergerObservor ==
  Valpha : Inport
  Vbeta : Inport  Port=2
  Ialpha : Inport  Port=3
  Ibeta : Inport  Port=4
  We : Inport  Port=5
  Delay One Step : Delay  DelayLength=1  InitialCondition=single(0)
  Terminator : Terminator
  getE : Subsystem
  getSpeedandTheta : Subsystem
  Speed : Outport
  Theta : Outport  Port=2
  wires:
  getSpeedandTheta/2(Theta) -> Theta/1
  getSpeedandTheta/1(Speed) -> Speed/1
  getE/2(Ebeta) -> getSpeedandTheta/2(Ebeta)
  getE/1(Ealpha) -> getSpeedandTheta/1(Ealpha)
  Ibeta/1 -> getE/4(Ibeta)
  Ialpha/1 -> getE/3(Ialpha)
  Vbeta/1 -> getE/2(Vbeta)
  Valpha/1 -> getE/1(Valpha)
  getSpeedandTheta/3(We) -> Delay One Step/1
  We/1 -> Terminator/1
  Delay One Step/1 -> getE/5(We)

== system BLAC_MotorCtrl_Math/HFTask/axisTransform ==
  Ia : Inport
  Ib : Inport  Port=2
  SinTheta : Inport  Port=3
  CosTheta : Inport  Port=4
  Add1 : Sum
  Product{,1..3} (4 alike) : Product
  Signal Copy : SignalConversion  OverrideOpt=off
  Subtract : Sum  Inputs=-+
  a_plus_2b : Sum  Inputs=+++  RndMeth=Simplest  OutDataTypeStr=Inherit: Same as first input
  one_by_sqrt3 : Gain  Gain=1/sqrt(3)  RndMeth=Simplest  OutDataTypeStr=Inherit: Same as input
  Ialpha : Outport
  Ibeta : Outport  Port=2
  Id : Outport  Port=3
  Iq : Outport  Port=4
  wires:
  Product3/1 -> Subtract/2
  Product2/1 -> Subtract/1
  Add1/1 -> Id/1  "Id"
  Subtract/1 -> Iq/1  "Iq"
  Product/1 -> Add1/1
  Product1/1 -> Add1/2
  CosTheta/1 -> Product3/2, Product/2
  SinTheta/1 -> Product2/2, Product1/2
  a_plus_2b/1 -> one_by_sqrt3/1
  one_by_sqrt3/1 -> Ibeta/1, Product3/1, Product1/1  "Ibeta"
  Signal Copy/1 -> Ialpha/1, Product2/1, Product/1  "Ialpha"
  Ia/1 -> a_plus_2b/1, Signal Copy/1
  Ib/1 -> a_plus_2b/3, a_plus_2b/2

== system BLAC_MotorCtrl_Math/HFTask/currentADRC ==
  note: ADRC开发日志:
      | 20251229：
      | 感觉观测器参数存在问题，观测值瞬间会和参考值相等，导致PI控制器调节电流增速较慢
      | 2026.01.05
      | 1、LESO中的两个fal函数出现周期性震荡
      | 2、NLSEF中的电压输出值只有1.xV，电机转速无法提升
      | 2026.01.07
      | 1、减小NLSEF的参数，可以实现系统的收敛，且效果与PI控制器类似
  IdRef : Inport
  IqRef : Inport  Port=2
  Id : Inport  Port=3
  Iq : Inport  Port=4
  Ud : Inport  Port=5
  Uq : Inport  Port=6
  IntregralResetFlag : Inport  Port=7
  Wm : Inport  Port=8
  Delay One Step : Delay  InitialCondition=single(0)
  Delay One Step1 : Delay  InitialCondition=single(0)
  LESO : Subsystem  VariantControl=ESO
  NLSEF : Subsystem  VariantControl=NLSEF
  Terminator : Terminator
  UdRef : Outport
  UqRef : Outport  Port=2
  wires:
  NLSEF/1(Ud_ADRC) -> UdRef/1  "UdRef"
  NLSEF/2(Uq_ADRC) -> UqRef/1  "UqRef"
  IdRef/1 -> NLSEF/1(Id_Ref)
  Id/1 -> LESO/1(Id)
  IqRef/1 -> NLSEF/2(Iq_Ref)
  Iq/1 -> LESO/3(Iq)
  IntregralResetFlag/1 -> Terminator/1
  Delay One Step/1 -> LESO/2(Ud)
  Delay One Step1/1 -> LESO/4(Uq)
  LESO/2(Iq_ESO) -> NLSEF/4(Iq_ESO)
  LESO/1(Id_ESO) -> NLSEF/3(Id_ESO)
  LESO/3(Id_Dis) -> NLSEF/5(Id_ESO_Dis)
  LESO/4(Iq_Dis) -> NLSEF/6(Iq_ESO_Dis)
  Ud/1 -> Delay One Step/1
  Uq/1 -> Delay One Step1/1

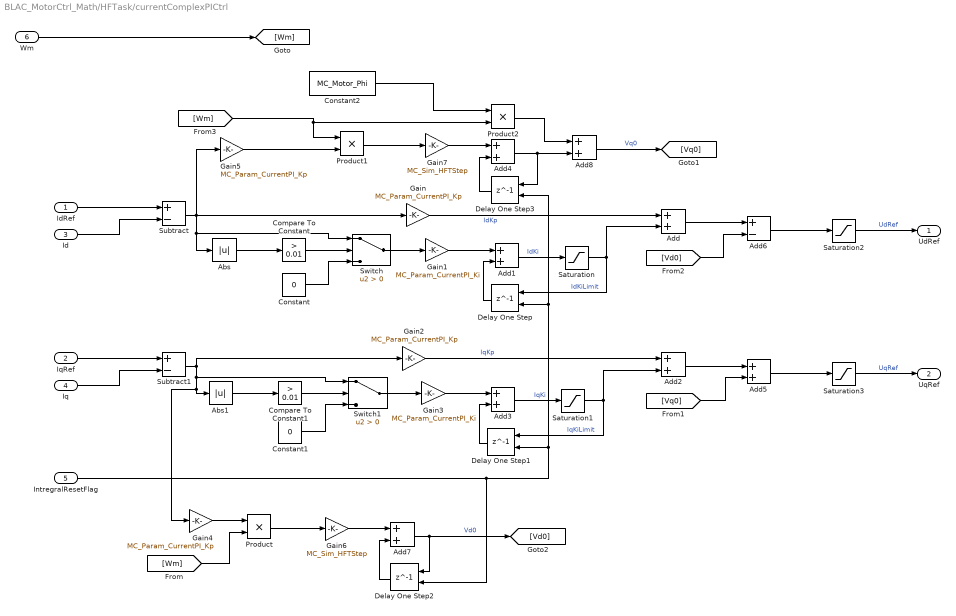
== system BLAC_MotorCtrl_Math/HFTask/currentComplexPICtrl ==
  IdRef : Inport
  IqRef : Inport  Port=2
  Id : Inport  Port=3
  Iq : Inport  Port=4
  IntregralResetFlag : Inport  Port=5
  Wm : Inport  Port=6
  Abs : Abs  SaturateOnIntegerOverflow=off
  Abs1 : Abs  SaturateOnIntegerOverflow=off
  Add{,2,5,8} (4 alike) : Sum
  Add{1,3..4,7} (4 alike) : Sum  OutDataTypeStr=single
  Add6 : Sum  Inputs=+-
  Compare To Constant : simulink/Logic and Bit Operations/Compare To Constant  relop=>  const=0.01  OutDataTypeStr=boolean
  Compare To Constant1 : simulink/Logic and Bit Operations/Compare To Constant  relop=>  const=0.01  OutDataTypeStr=boolean
  Constant : Constant  Value=0  OutDataTypeStr=single
  Constant1 : Constant  Value=0  OutDataTypeStr=single
  Constant2 : Constant  Value=MC_Motor_Phi  OutDataTypeStr=single
  Delay One Step{,1..3} (4 alike) : Delay  DelayLength=1  ExternalReset=Level
      settings: InputPortMap=u0,r5
  Gain : Gain  Gain=MC_Param_CurrentPI_Kp  OutDataTypeStr=single
  Gain1 : Gain  Gain=MC_Param_CurrentPI_Ki  OutDataTypeStr=single
  Gain2 : Gain  Gain=MC_Param_CurrentPI_Kp  OutDataTypeStr=single
  Gain3 : Gain  Gain=MC_Param_CurrentPI_Ki  OutDataTypeStr=single
  Gain4 : Gain  Gain=MC_Param_CurrentPI_Kp
  Gain5 : Gain  Gain=MC_Param_CurrentPI_Kp
  Gain6 : Gain  Gain=MC_Sim_HFTStep  OutDataTypeStr=single
  Gain7 : Gain  Gain=MC_Sim_HFTStep  OutDataTypeStr=single
  Product : Product
  Product1 : Product
  Product2 : Product
  Saturation : Saturate  UpperLimit=MC_Param_CurrentPI_UdInteMax  LowerLimit=MC_Param_CurrentPI_UdInteMin
  Saturation1 : Saturate  UpperLimit=MC_Param_CurrentPI_UqInteMax  LowerLimit=MC_Param_CurrentPI_UqInteMin
  Saturation2 : Saturate  UpperLimit=MC_Param_CurrentPI_UdMax  LowerLimit=MC_Param_CurrentPI_UdMin
  Saturation3 : Saturate  UpperLimit=MC_Param_CurrentPI_UqMax  LowerLimit=MC_Param_CurrentPI_UqMin
  Subtract : Sum  Inputs=+-
  Subtract1 : Sum  Inputs=+-
  Switch : Switch  Criteria=u2 > Threshold  SaturateOnIntegerOverflow=off  InputSameDT=off
  Switch1 : Switch  Criteria=u2 > Threshold  SaturateOnIntegerOverflow=off  InputSameDT=off
  UdRef : Outport
  UqRef : Outport  Port=2
  wires:
  Wm/1 -> [Wm]
  Saturation3/1 -> UqRef/1  "UqRef"
  Saturation2/1 -> UdRef/1  "UdRef"
  [Vd0] -> Add6/2
  Add6/1 -> Saturation2/1
  Add/1 -> Add6/1
  [Vq0] -> Add5/2
  Add2/1 -> Add5/1
  [Wm] -> Product/2
  Id/1 -> Subtract/2
  Gain4/1 -> Product/1
  Switch1/1 -> Gain3/1
  Abs1/1 -> Compare To Constant1/1
  Compare To Constant1/1 -> Switch1/2
  Constant1/1 -> Switch1/3
  Constant/1 -> Switch/3
  Compare To Constant/1 -> Switch/2
  Switch/1 -> Gain1/1
  Add5/1 -> Saturation3/1
  IqRef/1 -> Subtract1/1
  Iq/1 -> Subtract1/2
  Subtract1/1 -> Gain2/1, Gain4/1, Abs1/1, Switch1/1
  Gain2/1 -> Add2/1  "IqKp"
  Gain3/1 -> Add3/1
  Delay One Step1/1 -> Add3/2
  Add3/1 -> Saturation1/1  "IqKi"
  Saturation1/1 -> Add2/2, Delay One Step1/1  "IqKiLimit"
  Saturation/1 -> Delay One Step/1, Add/2  "IdKiLimit"
  Add1/1 -> Saturation/1  "IdKi"
  Delay One Step/1 -> Add1/2
  Gain1/1 -> Add1/1
  Abs/1 -> Compare To Constant/1
  Gain/1 -> Add/1  "IdKp"
  Subtract/1 -> Gain5/1, Abs/1, Switch/1, Gain/1
  IdRef/1 -> Subtract/1
  Gain6/1 -> Add7/1
  Product/1 -> Gain6/1
  Delay One Step2/1 -> Add7/2
  Add7/1 -> [Vd0], Delay One Step2/1  "Vd0"
  Add4/1 -> Delay One Step3/1, Add8/2
  Delay One Step3/1 -> Add4/2
  Gain7/1 -> Add4/1
  IntregralResetFlag/1 -> Delay One Step2/2, Delay One Step1/2, Delay One Step3/2, Delay One Step/2
  Product1/1 -> Gain7/1
  Constant2/1 -> Product2/1
  Gain5/1 -> Product1/2
  Add8/1 -> [Vq0]  "Vq0"
  Product2/1 -> Add8/1
  [Wm] -> Product1/1, Product2/2

== system BLAC_MotorCtrl_Math/HFTask/currentDBC ==
  note: 无差拍电流控制器（延时1拍）
  IdRef : Inport
  IqRef : Inport  Port=2
  Id : Inport  Port=3
  Iq : Inport  Port=4
  Wm : Inport  Port=5
  Add5 : Sum  Inputs=++-
  Add6 : Sum  Inputs=+++
  Add7 : Sum
  Constant1 : Constant  Value=MC_Motor_Phi  OutDataTypeStr=single
  Gain10 : Gain  Gain=MC_Motor_Stator_Lq
  Gain11 : Gain  Gain=MC_Motor_Stator_Lq/MC_Sim_HFTStep
  Gain12 : Gain  Gain=MC_Motor_Stator_Rs-(MC_Motor_Stator_Lq/MC_Sim_HFTStep)
  Gain13 : Gain  Gain=MC_Motor_Stator_Ld
  Gain8 : Gain  Gain=MC_Motor_Stator_Ld/MC_Sim_HFTStep
  Gain9 : Gain  Gain=MC_Motor_Stator_Rs-(MC_Motor_Stator_Ld/MC_Sim_HFTStep)
  Product2 : Product
  Product3 : Product
  Saturation : Saturate  UpperLimit=MC_Param_CurrentPI_UdMax  LowerLimit=MC_Param_CurrentPI_UdMin
  Saturation1 : Saturate  UpperLimit=MC_Param_CurrentPI_UqMax  LowerLimit=MC_Param_CurrentPI_UqMin
  UdRef : Outport
  UqRef : Outport  Port=2
  wires:
  Wm/1 -> [Wm]
  Iq/1 -> [Iq]
  Id/1 -> [Id]
  IqRef/1 -> [IqRef]
  IdRef/1 -> [IdRef]
  [IdRef] -> Gain8/1
  Gain8/1 -> Add5/1  "IdRef_Vd"
  [Id] -> Gain9/1
  Gain9/1 -> Add5/2  "Id_Vd"
  [Iq] -> Gain10/1
  Gain10/1 -> Product2/2
  [Wm] -> Product2/1
  [IqRef] -> Gain11/1
  Gain11/1 -> Add6/1  "IqRef_Vq"
  Gain12/1 -> Add6/2  "Iq_Vq"
  [Iq] -> Gain12/1
  [Wm] -> Product3/1
  Add7/1 -> Product3/2
  Constant1/1 -> Add7/2
  Gain13/1 -> Add7/1
  [Id] -> Gain13/1
  Saturation/1 -> UdRef/1  "UdRef_DBC"
  Saturation1/1 -> UqRef/1  "UqRef_DBC"
  Add5/1 -> Saturation/1
  Product2/1 -> Add5/3  "Iq_Vd"
  Add6/1 -> Saturation1/1
  Product3/1 -> Add6/3  "Id_Vq"

== system BLAC_MotorCtrl_Math/HFTask/currentPIControl ==
  IdRef : Inport
  IqRef : Inport  Port=2
  Id : Inport  Port=3
  Iq : Inport  Port=4
  IntregralResetFlag : Inport  Port=5
  Wm : Inport  Port=6
  Abs : Abs  SaturateOnIntegerOverflow=off
  Abs1 : Abs  SaturateOnIntegerOverflow=off
  Add{,2,4..5} (4 alike) : Sum
  Add1 : Sum  OutDataTypeStr=single
  Add3 : Sum  OutDataTypeStr=single
  Add6 : Sum  Inputs=+-
  Compare To Constant : simulink/Logic and Bit Operations/Compare To Constant  relop=>  const=0.01  OutDataTypeStr=boolean
  Compare To Constant1 : simulink/Logic and Bit Operations/Compare To Constant  relop=>  const=0.01  OutDataTypeStr=boolean
  Constant : Constant  Value=0  OutDataTypeStr=single
  Constant1 : Constant  Value=0  OutDataTypeStr=single
  Constant2 : Constant  Value=MC_Motor_Phi  OutDataTypeStr=single
  Delay One Step : Delay  DelayLength=1  ExternalReset=Level
      settings: InputPortMap=u0,r5
  Delay One Step1 : Delay  DelayLength=1  ExternalReset=Level
      settings: InputPortMap=u0,r5
  Gain : Gain  Gain=MC_Param_CurrentPI_Kp  OutDataTypeStr=single
  Gain1 : Gain  Gain=MC_Param_CurrentPI_Ki  OutDataTypeStr=single
  Gain2 : Gain  Gain=MC_Param_CurrentPI_Kp  OutDataTypeStr=single
  Gain3 : Gain  Gain=MC_Param_CurrentPI_Ki  OutDataTypeStr=single
  Gain4 : Gain  Gain=MC_Motor_Stator_Lq
  Gain5 : Gain  Gain=MC_Motor_Stator_Ld
  Product : Product
  Product1 : Product
  Saturation : Saturate  UpperLimit=MC_Param_CurrentPI_UdInteMax  LowerLimit=MC_Param_CurrentPI_UdInteMin
  Saturation1 : Saturate  UpperLimit=MC_Param_CurrentPI_UqInteMax  LowerLimit=MC_Param_CurrentPI_UqInteMin
  Saturation2 : Saturate  UpperLimit=MC_Param_CurrentPI_UdMax  LowerLimit=MC_Param_CurrentPI_UdMin
  Saturation3 : Saturate  UpperLimit=MC_Param_CurrentPI_UqMax  LowerLimit=MC_Param_CurrentPI_UqMin
  Subtract : Sum  Inputs=+-
  Subtract1 : Sum  Inputs=+-
  Switch : Switch  Criteria=u2 > Threshold  SaturateOnIntegerOverflow=off  InputSameDT=off
  Switch1 : Switch  Criteria=u2 > Threshold  SaturateOnIntegerOverflow=off  InputSameDT=off
  UdRef : Outport
  UqRef : Outport  Port=2
  wires:
  IdRef/1 -> Subtract/1
  Subtract/1 -> Gain/1, Switch/1, Abs/1
  Gain/1 -> Add/1  "IdKp"
  Abs/1 -> Compare To Constant/1
  Gain1/1 -> Add1/1
  Delay One Step/1 -> Add1/2
  Add1/1 -> Saturation/1  "IdKi"
  Saturation/1 -> Add/2, Delay One Step/1  "IdKiLimit"
  Saturation1/1 -> Delay One Step1/1, Add2/2  "IqKiLimit"
  Add3/1 -> Saturation1/1  "IqKi"
  Delay One Step1/1 -> Add3/2
  Gain3/1 -> Add3/1
  Gain2/1 -> Add2/1  "IqKp"
  Subtract1/1 -> Switch1/1, Abs1/1, Gain2/1
  Iq/1 -> Gain4/1, Subtract1/2
  IqRef/1 -> Subtract1/1
  IntregralResetFlag/1 -> Delay One Step/2, Delay One Step1/2
  Add5/1 -> Saturation3/1
  Switch/1 -> Gain1/1
  Compare To Constant/1 -> Switch/2
  Constant/1 -> Switch/3
  Constant1/1 -> Switch1/3
  Compare To Constant1/1 -> Switch1/2
  Abs1/1 -> Compare To Constant1/1
  Switch1/1 -> Gain3/1
  Gain4/1 -> Product/1
  Id/1 -> Gain5/1, Subtract/2
  [Wm] -> Product/2
  Gain5/1 -> Add4/1
  Add4/1 -> Product1/2
  Constant2/1 -> Add4/2
  Product1/1 -> [Vq0]
  Product/1 -> [Vd0]
  Add2/1 -> Add5/1
  [Vq0] -> Add5/2
  Add/1 -> Add6/1
  Add6/1 -> Saturation2/1
  [Vd0] -> Add6/2
  Saturation2/1 -> UdRef/1  "UdRef"
  Saturation3/1 -> UqRef/1  "UqRef"
  [Wm] -> Product1/1
  Wm/1 -> [Wm]

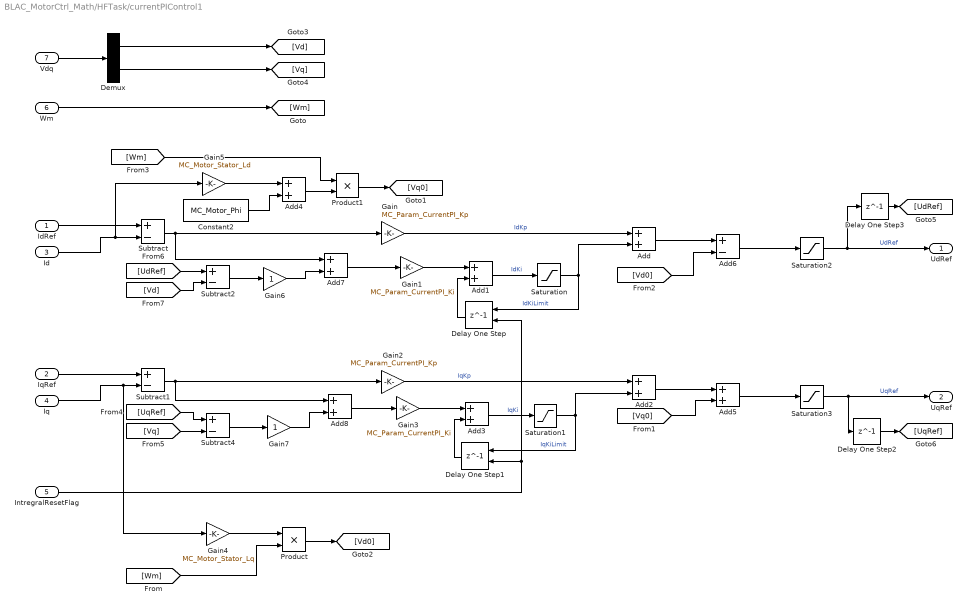
== system BLAC_MotorCtrl_Math/HFTask/currentPIControl1 ==
  IdRef : Inport
  IqRef : Inport  Port=2
  Id : Inport  Port=3
  Iq : Inport  Port=4
  IntregralResetFlag : Inport  Port=5
  Wm : Inport  Port=6
  Vdq : Inport  Port=7
  Add{,2,4..5,7..8} (6 alike) : Sum
  Add1 : Sum  OutDataTypeStr=single
  Add3 : Sum  OutDataTypeStr=single
  Add6 : Sum  Inputs=+-
  Constant2 : Constant  Value=MC_Motor_Phi  OutDataTypeStr=single
  Delay One Step : Delay  DelayLength=1  ExternalReset=Level
      settings: InputPortMap=u0,r5
  Delay One Step1 : Delay  DelayLength=1  ExternalReset=Level
      settings: InputPortMap=u0,r5
  Delay One Step2 : Delay  DelayLength=1  InitialCondition=single(0)
  Delay One Step3 : Delay  DelayLength=1  InitialCondition=single(0)
  Demux : Demux  Outputs=2
  Gain : Gain  Gain=MC_Param_CurrentPI_Kp  OutDataTypeStr=single
  Gain1 : Gain  Gain=MC_Param_CurrentPI_Ki  OutDataTypeStr=single
  Gain2 : Gain  Gain=MC_Param_CurrentPI_Kp  OutDataTypeStr=single
  Gain3 : Gain  Gain=MC_Param_CurrentPI_Ki  OutDataTypeStr=single
  Gain4 : Gain  Gain=MC_Motor_Stator_Lq
  Gain5 : Gain  Gain=MC_Motor_Stator_Ld
  Gain6 : Gain
  Gain7 : Gain
  Product : Product
  Product1 : Product
  Saturation : Saturate  UpperLimit=MC_Param_CurrentPI_UdInteMax  LowerLimit=MC_Param_CurrentPI_UdInteMin
  Saturation1 : Saturate  UpperLimit=MC_Param_CurrentPI_UqInteMax  LowerLimit=MC_Param_CurrentPI_UqInteMin
  Saturation2 : Saturate  UpperLimit=MC_Param_CurrentPI_UdMax  LowerLimit=MC_Param_CurrentPI_UdMin
  Saturation3 : Saturate  UpperLimit=MC_Param_CurrentPI_UqMax  LowerLimit=MC_Param_CurrentPI_UqMin
  Subtract{,1..2,4} (4 alike) : Sum  Inputs=+-
  UdRef : Outport
  UqRef : Outport  Port=2
  wires:
  Wm/1 -> [Wm]
  [Wm] -> Product1/1
  Saturation3/1 -> Delay One Step2/1, UqRef/1  "UqRef"
  Saturation2/1 -> Delay One Step3/1, UdRef/1  "UdRef"
  [Vd0] -> Add6/2
  Add6/1 -> Saturation2/1
  Add/1 -> Add6/1
  [Vq0] -> Add5/2
  Add2/1 -> Add5/1
  Product/1 -> [Vd0]
  Product1/1 -> [Vq0]
  Constant2/1 -> Add4/2
  Add4/1 -> Product1/2
  Gain5/1 -> Add4/1
  [Wm] -> Product/2
  Id/1 -> Subtract/2, Gain5/1
  Gain4/1 -> Product/1
  Add8/1 -> Gain3/1
  Add5/1 -> Saturation3/1
  IntregralResetFlag/1 -> Delay One Step1/2, Delay One Step/2
  IqRef/1 -> Subtract1/1
  Iq/1 -> Subtract1/2, Gain4/1
  Subtract1/1 -> Add8/1, Gain2/1
  Gain2/1 -> Add2/1  "IqKp"
  Gain3/1 -> Add3/1
  Delay One Step1/1 -> Add3/2
  Add3/1 -> Saturation1/1  "IqKi"
  Saturation1/1 -> Add2/2, Delay One Step1/1  "IqKiLimit"
  Saturation/1 -> Delay One Step/1, Add/2  "IdKiLimit"
  Add1/1 -> Saturation/1  "IdKi"
  Delay One Step/1 -> Add1/2
  Gain1/1 -> Add1/1
  Gain/1 -> Add/1  "IdKp"
  Subtract/1 -> Add7/1, Gain/1
  IdRef/1 -> Subtract/1
  Vdq/1 -> Demux/1
  Demux/1 -> [Vd]
  Demux/2 -> [Vq]
  Add7/1 -> Gain1/1
  [Vq] -> Subtract4/2
  [UqRef] -> Subtract4/1
  Subtract2/1 -> Gain6/1
  Gain6/1 -> Add7/2
  Subtract4/1 -> Gain7/1
  Gain7/1 -> Add8/2
  [UdRef] -> Subtract2/1
  [Vd] -> Subtract2/2
  Delay One Step2/1 -> [UqRef]
  Delay One Step3/1 -> [UdRef]

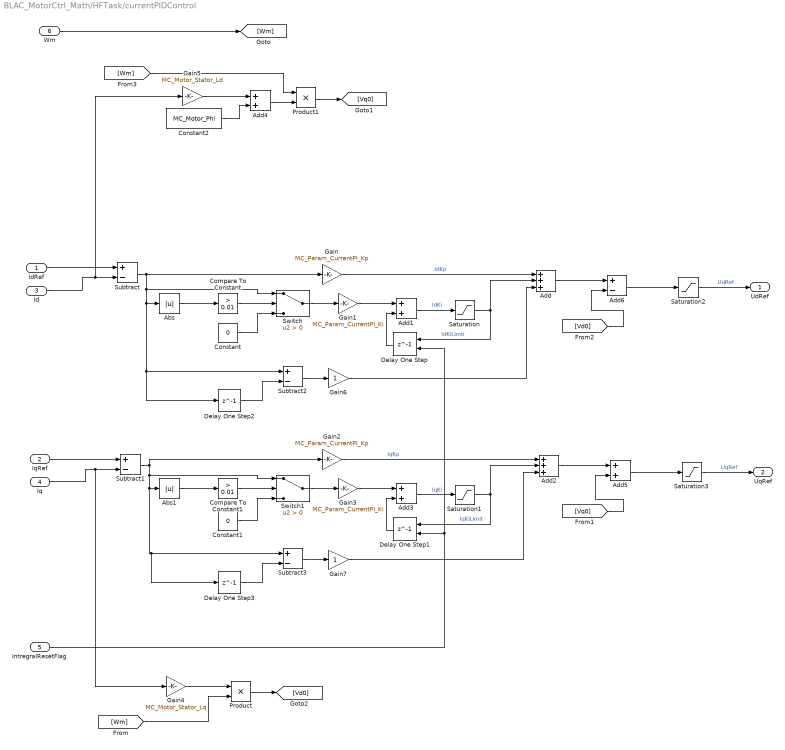
== system BLAC_MotorCtrl_Math/HFTask/currentPIDControl ==
  IdRef : Inport
  IqRef : Inport  Port=2
  Id : Inport  Port=3
  Iq : Inport  Port=4
  IntregralResetFlag : Inport  Port=5
  Wm : Inport  Port=6
  Abs : Abs  SaturateOnIntegerOverflow=off
  Abs1 : Abs  SaturateOnIntegerOverflow=off
  Add : Sum  Inputs=+++
  Add1 : Sum  OutDataTypeStr=single
  Add2 : Sum  Inputs=+++
  Add3 : Sum  OutDataTypeStr=single
  Add4 : Sum
  Add5 : Sum
  Add6 : Sum  Inputs=+-
  Compare To Constant : simulink/Logic and Bit Operations/Compare To Constant  relop=>  const=0.01  OutDataTypeStr=boolean
  Compare To Constant1 : simulink/Logic and Bit Operations/Compare To Constant  relop=>  const=0.01  OutDataTypeStr=boolean
  Constant : Constant  Value=0  OutDataTypeStr=single
  Constant1 : Constant  Value=0  OutDataTypeStr=single
  Constant2 : Constant  Value=MC_Motor_Phi  OutDataTypeStr=single
  Delay One Step : Delay  DelayLength=1  ExternalReset=Level
      settings: InputPortMap=u0,r5
  Delay One Step1 : Delay  DelayLength=1  ExternalReset=Level
      settings: InputPortMap=u0,r5
  Delay One Step2 : Delay  DelayLength=1  InitialCondition=single(0)
  Delay One Step3 : Delay  DelayLength=1  InitialCondition=single(0)
  Gain : Gain  Gain=MC_Param_CurrentPI_Kp  OutDataTypeStr=single
  Gain1 : Gain  Gain=MC_Param_CurrentPI_Ki  OutDataTypeStr=single
  Gain2 : Gain  Gain=MC_Param_CurrentPI_Kp  OutDataTypeStr=single
  Gain3 : Gain  Gain=MC_Param_CurrentPI_Ki  OutDataTypeStr=single
  Gain4 : Gain  Gain=MC_Motor_Stator_Lq
  Gain5 : Gain  Gain=MC_Motor_Stator_Ld
  Gain6 : Gain
  Gain7 : Gain
  Product : Product
  Product1 : Product
  Saturation : Saturate  UpperLimit=MC_Param_CurrentPI_UdInteMax  LowerLimit=MC_Param_CurrentPI_UdInteMin
  Saturation1 : Saturate  UpperLimit=MC_Param_CurrentPI_UqInteMax  LowerLimit=MC_Param_CurrentPI_UqInteMin
  Saturation2 : Saturate  UpperLimit=MC_Param_CurrentPI_UdMax  LowerLimit=MC_Param_CurrentPI_UdMin
  Saturation3 : Saturate  UpperLimit=MC_Param_CurrentPI_UqMax  LowerLimit=MC_Param_CurrentPI_UqMin
  Subtract{,1..3} (4 alike) : Sum  Inputs=+-
  Switch : Switch  Criteria=u2 > Threshold  SaturateOnIntegerOverflow=off  InputSameDT=off
  Switch1 : Switch  Criteria=u2 > Threshold  SaturateOnIntegerOverflow=off  InputSameDT=off
  UdRef : Outport
  UqRef : Outport  Port=2
  wires:
  IdRef/1 -> Subtract/1
  Subtract/1 -> Gain/1, Switch/1, Subtract2/1, Delay One Step2/1, Abs/1
  Gain/1 -> Add/1  "IdKp"
  Abs/1 -> Compare To Constant/1
  Gain1/1 -> Add1/1
  Delay One Step/1 -> Add1/2
  Add1/1 -> Saturation/1  "IdKi"
  Saturation/1 -> Add/2, Delay One Step/1  "IdKiLimit"
  Saturation1/1 -> Delay One Step1/1, Add2/2  "IqKiLimit"
  Add3/1 -> Saturation1/1  "IqKi"
  Delay One Step1/1 -> Add3/2
  Gain3/1 -> Add3/1
  Gain2/1 -> Add2/1  "IqKp"
  Iq/1 -> Subtract1/2, Gain4/1
  IqRef/1 -> Subtract1/1
  IntregralResetFlag/1 -> Delay One Step/2, Delay One Step1/2
  Add5/1 -> Saturation3/1
  Switch/1 -> Gain1/1
  Compare To Constant/1 -> Switch/2
  Constant/1 -> Switch/3
  Constant1/1 -> Switch1/3
  Compare To Constant1/1 -> Switch1/2
  Abs1/1 -> Compare To Constant1/1
  Switch1/1 -> Gain3/1
  Gain4/1 -> Product/1
  Id/1 -> Gain5/1, Subtract/2
  [Wm] -> Product/2
  Gain5/1 -> Add4/1
  Add4/1 -> Product1/2
  Constant2/1 -> Add4/2
  Product1/1 -> [Vq0]
  Product/1 -> [Vd0]
  Add2/1 -> Add5/1
  [Vq0] -> Add5/2
  Add/1 -> Add6/1
  Add6/1 -> Saturation2/1
  [Vd0] -> Add6/2
  Saturation2/1 -> UdRef/1  "UdRef"
  Saturation3/1 -> UqRef/1  "UqRef"
  [Wm] -> Product1/1
  Wm/1 -> [Wm]
  Delay One Step2/1 -> Subtract2/2
  Subtract2/1 -> Gain6/1
  Gain6/1 -> Add/3
  Gain7/1 -> Add2/3
  Subtract3/1 -> Gain7/1
  Delay One Step3/1 -> Subtract3/2
  Subtract1/1 -> Switch1/1, Delay One Step3/1, Subtract3/1, Abs1/1, Gain2/1

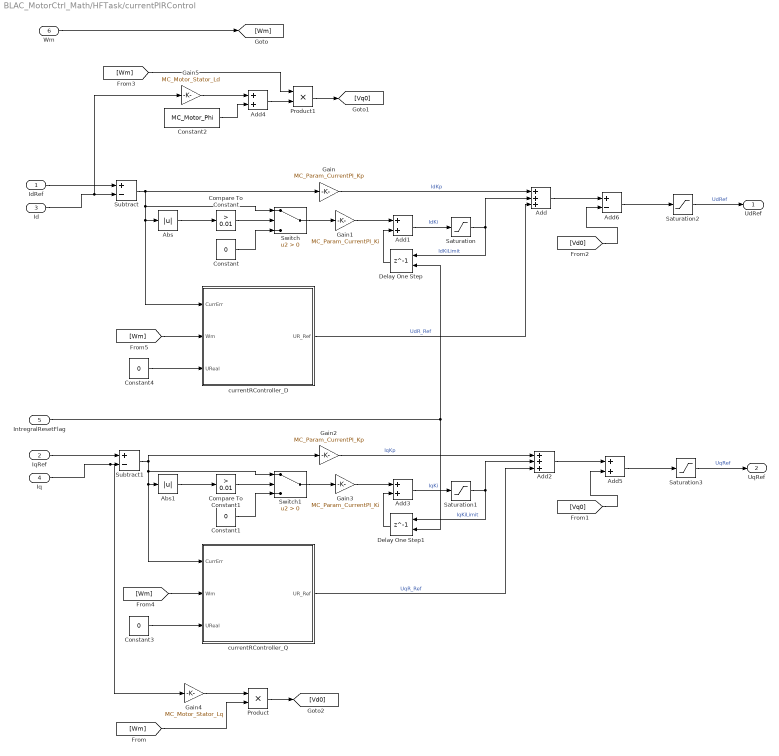
== system BLAC_MotorCtrl_Math/HFTask/currentPIRControl ==
  IdRef : Inport
  IqRef : Inport  Port=2
  Id : Inport  Port=3
  Iq : Inport  Port=4
  IntregralResetFlag : Inport  Port=5
  Wm : Inport  Port=6
  Abs : Abs  SaturateOnIntegerOverflow=off
  Abs1 : Abs  SaturateOnIntegerOverflow=off
  Add : Sum  Inputs=+++
  Add1 : Sum  OutDataTypeStr=single
  Add2 : Sum  Inputs=+++
  Add3 : Sum  OutDataTypeStr=single
  Add4 : Sum
  Add5 : Sum
  Add6 : Sum  Inputs=+-
  Compare To Constant : simulink/Logic and Bit Operations/Compare To Constant  relop=>  const=0.01  OutDataTypeStr=boolean
  Compare To Constant1 : simulink/Logic and Bit Operations/Compare To Constant  relop=>  const=0.01  OutDataTypeStr=boolean
  Constant{,1,3..4} (4 alike) : Constant  Value=0  OutDataTypeStr=single
  Constant2 : Constant  Value=MC_Motor_Phi  OutDataTypeStr=single
  Delay One Step : Delay  DelayLength=1  ExternalReset=Level
      settings: InputPortMap=u0,r5
  Delay One Step1 : Delay  DelayLength=1  ExternalReset=Level
      settings: InputPortMap=u0,r5
  Gain : Gain  Gain=MC_Param_CurrentPI_Kp  OutDataTypeStr=single
  Gain1 : Gain  Gain=MC_Param_CurrentPI_Ki  OutDataTypeStr=single
  Gain2 : Gain  Gain=MC_Param_CurrentPI_Kp  OutDataTypeStr=single
  Gain3 : Gain  Gain=MC_Param_CurrentPI_Ki  OutDataTypeStr=single
  Gain4 : Gain  Gain=MC_Motor_Stator_Lq
  Gain5 : Gain  Gain=MC_Motor_Stator_Ld
  Product : Product
  Product1 : Product
  Saturation : Saturate  UpperLimit=MC_Param_CurrentPI_UdInteMax  LowerLimit=MC_Param_CurrentPI_UdInteMin
  Saturation1 : Saturate  UpperLimit=MC_Param_CurrentPI_UqInteMax  LowerLimit=MC_Param_CurrentPI_UqInteMin
  Saturation2 : Saturate  UpperLimit=MC_Param_CurrentPI_UdMax  LowerLimit=MC_Param_CurrentPI_UdMin
  Saturation3 : Saturate  UpperLimit=MC_Param_CurrentPI_UqMax  LowerLimit=MC_Param_CurrentPI_UqMin
  Subtract : Sum  Inputs=+-
  Subtract1 : Sum  Inputs=+-
  Switch : Switch  Criteria=u2 > Threshold  SaturateOnIntegerOverflow=off  InputSameDT=off
  Switch1 : Switch  Criteria=u2 > Threshold  SaturateOnIntegerOverflow=off  InputSameDT=off
  currentRController_D : Subsystem
  currentRController_Q : Subsystem
  UdRef : Outport
  UqRef : Outport  Port=2
  wires:
  Subtract1/1 -> Gain2/1, currentRController_Q/1(CurrErr), Abs1/1, Switch1/1
  Wm/1 -> [Wm]
  [Wm] -> Product1/1
  Saturation3/1 -> UqRef/1  "UqRef"
  Saturation2/1 -> UdRef/1  "UdRef"
  [Vd0] -> Add6/2
  Add6/1 -> Saturation2/1
  Add/1 -> Add6/1
  [Vq0] -> Add5/2
  Add2/1 -> Add5/1
  Product/1 -> [Vd0]
  Product1/1 -> [Vq0]
  Constant2/1 -> Add4/2
  Add4/1 -> Product1/2
  Gain5/1 -> Add4/1
  [Wm] -> Product/2
  Id/1 -> Subtract/2, Gain5/1
  Gain4/1 -> Product/1
  Switch1/1 -> Gain3/1
  Abs1/1 -> Compare To Constant1/1
  Compare To Constant1/1 -> Switch1/2
  Constant1/1 -> Switch1/3
  Constant/1 -> Switch/3
  Compare To Constant/1 -> Switch/2
  Switch/1 -> Gain1/1
  Add5/1 -> Saturation3/1
  IntregralResetFlag/1 -> Delay One Step1/2, Delay One Step/2
  IqRef/1 -> Subtract1/1
  Iq/1 -> Gain4/1, Subtract1/2
  Gain2/1 -> Add2/1  "IqKp"
  Gain3/1 -> Add3/1
  Delay One Step1/1 -> Add3/2
  Add3/1 -> Saturation1/1  "IqKi"
  Saturation1/1 -> Add2/2, Delay One Step1/1  "IqKiLimit"
  Saturation/1 -> Delay One Step/1, Add/2  "IdKiLimit"
  Add1/1 -> Saturation/1  "IdKi"
  Delay One Step/1 -> Add1/2
  Gain1/1 -> Add1/1
  Abs/1 -> Compare To Constant/1
  Gain/1 -> Add/1  "IdKp"
  Subtract/1 -> currentRController_D/1(CurrErr), Abs/1, Switch/1, Gain/1
  IdRef/1 -> Subtract/1
  currentRController_D/1(UR_Ref) -> Add/3  "UdR_Ref"
  currentRController_Q/1(UR_Ref) -> Add2/3  "UqR_Ref"
  [Wm] -> currentRController_Q/2(Wm)
  Constant3/1 -> currentRController_Q/3(UReal)
  Constant4/1 -> currentRController_D/3(UReal)
  [Wm] -> currentRController_D/2(Wm)

== system BLAC_MotorCtrl_Math/HFTask/fluxobservor ==
  Valpha : Inport
  Vbeta : Inport  Port=2
  Ialpha : Inport  Port=3
  Ibeta : Inport  Port=4
  getFlux : Subsystem
  getSpeedandTheta : Subsystem
  Speed : Outport
  Theta : Outport  Port=2
  wires:
  getSpeedandTheta/2(Theta) -> Theta/1
  getSpeedandTheta/1(Speed) -> Speed/1
  getFlux/2(Phibeta) -> getSpeedandTheta/2(Phibeta)
  getFlux/1(Phialpha) -> getSpeedandTheta/1(Phialpha)
  Ibeta/1 -> getFlux/4(Ibeta)
  Ialpha/1 -> getFlux/3(Ialpha)
  Vbeta/1 -> getFlux/2(Vbeta)
  Valpha/1 -> getFlux/1(Valpha)

== system BLAC_MotorCtrl_Math/HFTask/getCurrentPredict ==
  note: 开发日志：
      | 2025.03.26:
      | 1、完成两节拍的电流预测
      | 2025.03.27：
      | 1、采用延时2个周期的采样电流和延时1个周期的设定电压进行延时1个周期的电机电流预测
  Ud1 : Inport
  Id : Inport  Port=2
  Uq1 : Inport  Port=3
  Iq : Inport  Port=4
  Wm : Inport  Port=5
  Add : Sum  Inputs=+++
  Add1 : Sum  Inputs=++-
  Add2 : Sum
  Constant : Constant  Value=MC_Motor_Phi  OutDataTypeStr=single
  Gain1 : Gain  Gain=MC_Sim_HFTStep/MC_Motor_Stator_Lq
  Gain4 : Gain  Gain=MC_Sim_HFTStep/MC_Motor_Stator_Ld
  Gain5 : Gain  Gain=1-(MC_Sim_HFTStep*MC_Motor_Stator_Rs/MC_Motor_Stator_Ld)
  Gain6 : Gain  Gain=MC_Sim_HFTStep/MC_Motor_Stator_Lq
  Gain7 : Gain  Gain=1-(MC_Sim_HFTStep*MC_Motor_Stator_Rs/MC_Motor_Stator_Lq)
  Gain8 : Gain  Gain=MC_Sim_HFTStep*MC_Motor_Stator_Ld/MC_Motor_Stator_Lq
  Gain9 : Gain  Gain=(MC_Sim_HFTStep*MC_Motor_Stator_Lq/MC_Motor_Stator_Ld)
  Product : Product
  Product1 : Product
  Id_Pre : Outport
  Iq_Pre : Outport  Port=2
  wires:
  [Iq] -> Gain7/1
  [Wm] -> Product1/1
  Iq/1 -> [Iq]
  Gain4/1 -> Add/1  "Ud_Id1"
  [Iq] -> Gain9/1
  [Uq1] -> Gain6/1
  Gain9/1 -> Product/1
  Constant/1 -> Gain1/1
  Product/1 -> Add/3  "Iq_Id1"
  [Ud1] -> Gain4/1
  Gain6/1 -> Add1/1  "Uq_Iq1"
  Gain7/1 -> Add1/2  "Iq_Iq1"
  Gain5/1 -> Add/2  "Id_Id1"
  [Id] -> Gain8/1
  Product1/1 -> Add1/3  "Id_Iq1"
  Gain8/1 -> Add2/1
  [Wm] -> Product/2
  Id/1 -> [Id]
  Add2/1 -> Product1/2
  [Id] -> Gain5/1
  Wm/1 -> [Wm]
  Gain1/1 -> Add2/2
  Add/1 -> Id_Pre/1  "Id1"
  Add1/1 -> Iq_Pre/1  "Iq1"
  Ud1/1 -> [Ud1]
  Uq1/1 -> [Uq1]
